simulink model "ponto2"  (R2016b)
settings: Solver=VariableStepAuto  StartTime=0.0  StopTime=500  RelTol=1e-3
values from neighbouring files (symbols this model uses):
  a = [xu xw -aa0*u0 -g*cos(tt0) ... (first row only)    [tb30.m]
  b = [xde xdt; zde 0; mde+mwp*zde mdt; 0 0]    [tb30.m]
  c = eye(4)    [tb30.m]
  d = zeros(4,2)    [tb30.m]
settings Model: Creator=inespassinhas  LastModifiedBy=inespassinhas

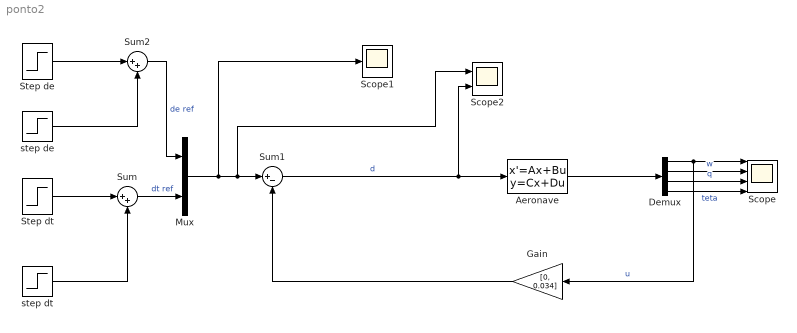
== system ponto2 ==
  Aeronave : StateSpace  A=a  B=b  C=c  D=d  X0=[0 0 0 0]
  Demux : Demux
  Gain : Gain  Gain=[0, 0.034]
  Mux : Mux  Inputs=2
  Scope : Scope  NumInputPorts=4
  Scope1 : Scope
  Scope2 : Scope  NumInputPorts=2
  Step de : Step  Time=200  After=0.1  SampleTime=40
  Step dt : Step  Time=10  After=0.1  SampleTime=10
  Sum : Sum  Inputs=|++
  Sum1 : Sum  Inputs=|+-
  Sum2 : Sum  Inputs=|++
  step de : Step  Time=250  After=-0.1  SampleTime=40
  step dt : Step  Time=80  After=-0.1  SampleTime=10
  wires:
  Aeronave/1 -> Demux/1
  Demux/1 -> Gain/1, Scope/1  "u"
  Demux/2 -> Scope/2  "w"
  Demux/3 -> Scope/3  "q"
  Demux/4 -> Scope/4  "teta"
  Step dt/1 -> Sum/1
  step dt/1 -> Sum/2
  step de/1 -> Sum2/2
  Step de/1 -> Sum2/1
  Sum2/1 -> Mux/1  "de ref"
  Sum/1 -> Mux/2  "dt ref"
  Gain/1 -> Sum1/2
  Mux/1 -> Scope1/1, Scope2/1, Sum1/1
  Sum1/1 -> Scope2/2, Aeronave/1  "d"
